simulink model "MBE_Simulation_04_Template_14_11_final"  (R2017b)
settings: Solver=FixedStepAuto  StartTime=0.0  StopTime=inf  FixedStep=0.05  RelTol=1e-3
libraries: simulink x67, canmsglib x4, instrumentlib x2, realtime_pacer_lib x1, hdlsllib x1
(part 3 of 4)

== system MBE_Simulation_04_Template_14_11_final/LeuchtenBlinkerBox/LB_Box_Simulation_Input/CanReceive_Cockpit_1 ==
  CanData_Cockpit_1_In : Inport
  Bus Selector : BusSelector  OutputSignals=CanData_Cockpit_1,CanTrigger_Cockpit_1
  Detect Change4 : simulink/Logic and Bit Operations/Detect Change  vinit=0  OutDataTypeStr=boolean
  Terminator6 : Terminator
  CanData_Cockpit_1_Out : Outport
  CanTrigger_Cockpit_1_Out : Outport  Port=2
  wires:
  Bus Selector/1 -> CanData_Cockpit_1_Out/1, Detect Change4/1  "<CanData_Cockpit_1>"
  Bus Selector/2 -> Terminator6/1  "<CanTrigger_Cockpit_1>"
  CanData_Cockpit_1_In/1 -> Bus Selector/1
  Detect Change4/1 -> CanTrigger_Cockpit_1_Out/1

== system MBE_Simulation_04_Template_14_11_final/LeuchtenBlinkerBox/LB_Box_Simulation_Input/CanReceive_Schloss_1 ==
  CanMsg_Schloss_1_In : Inport
  Bus Selector4 : BusSelector  OutputSignals=CanData_Schloss_1,CanTrigger_Schloss_1
  Detect Change4 : simulink/Logic and Bit Operations/Detect Change  vinit=0  OutDataTypeStr=boolean
  Terminator4 : Terminator
  CanData_Schloss_1_Out : Outport
  CanTrigger_Schloss_1_Out : Outport  Port=2
  wires:
  Bus Selector4/2 -> Terminator4/1  "<CanTrigger_Schloss_1>"
  CanMsg_Schloss_1_In/1 -> Bus Selector4/1
  Bus Selector4/1 -> Detect Change4/1, CanData_Schloss_1_Out/1  "<CanData_Schloss_1>"
  Detect Change4/1 -> CanTrigger_Schloss_1_Out/1

== system MBE_Simulation_04_Template_14_11_final/LeuchtenBlinkerBox/LB_Box_Simulation_Input/CanReceive_Sensor_1 ==
  CanMsg_Sensor_1_In : Inport
  Bus Selector2 : BusSelector  OutputSignals=CanData_Sensor_1,CanTrigger_Sensor_1
  CanData_Sensor_1_Out : Outport
  CanTrigger_Sensor_1_Out : Outport  Port=2
  wires:
  Bus Selector2/1 -> CanData_Sensor_1_Out/1  "<CanData_Sensor_1>"
  CanMsg_Sensor_1_In/1 -> Bus Selector2/1
  Bus Selector2/2 -> CanTrigger_Sensor_1_Out/1  "<CanTrigger_Sensor_1>"

== system MBE_Simulation_04_Template_14_11_final/LeuchtenBlinkerBox/LB_Box_Simulation_Input/GuiInput_LichtBox ==
  Bus Selector : BusSelector  OutputSignals=lightGenericButton
  GenericButton_Out : Outport
  wires:
  [lightInputBus] -> Bus Selector/1
  Bus Selector/1 -> GenericButton_Out/1  "<lightGenericButton>"

== system MBE_Simulation_04_Template_14_11_final/LeuchtenBlinkerBox/LB_Box_Simulation_Output/LeuchtenBlinkerLEDs ==
  FEL_LED : Inport  OutDataTypeStr=boolean
  ABL_LED : Inport  Port=2  OutDataTypeStr=boolean
  TFL_LED : Inport  Port=3  OutDataTypeStr=boolean
  BLL_LED : Inport  Port=4  OutDataTypeStr=boolean
  BLR_LED : Inport  Port=5  OutDataTypeStr=boolean
  BRL_LED : Inport  Port=6  OutDataTypeStr=boolean
  Terminator{,1..5} (6 alike) : Terminator
  wires:
  BLR_LED/1 -> Terminator1/1
  ABL_LED/1 -> Terminator3/1
  TFL_LED/1 -> Terminator2/1
  BLL_LED/1 -> Terminator/1
  FEL_LED/1 -> Terminator4/1
  BRL_LED/1 -> Terminator5/1

== system MBE_Simulation_04_Template_14_11_final/MLF-VirtualPlatform Setup/Subsystem/Triggered Subsystem ==
  outputAlarmSignals : Inport
  "outputLightSignals " : Inport  Port=2  OutDataTypeStr=boolean
  outputWindshieldSignals : Inport  Port=3  OutDataTypeStr=boolean
  Trigger : TriggerPort  TriggerType=falling  VariantControl=Variant
  Bus Selector : BusSelector  OutputSignals=lightUpperBeamHeadlight,lightReverselight,lightLowerBeamHeadlight,lightIndicatorRight,lightIndicatorLeft,lightGenericLightUp,lightGenericLightRight,lightGenericLightLeft,lightGenericLightDown,lightFoglightRight,lightFoglightLeft,lightDaylight,lightBrakelight,lightBacklight
  Bus Selector1 : BusSelector  OutputSignals=alarmLockLight,alarmGenericLightUp,alarmGenericLightRight,alarmGenericLightLeft,alarmGenericLightDown,alarmAlarmLight
  Bus Selector2 : BusSelector  OutputSignals=windshieldWiperD,windshieldWiperC,windshieldWiperB,windshieldWiperA,windshieldWasherPump,windshieldHeater,windshieldGenericLightUp,windshieldGenericLightRight,windshieldGenericLightLeft,windshieldGenericLightDown
  MATLAB Function : MATLAB Function  TreatAsAtomicUnit=on
  MATLAB Function1 : MATLAB Function  Commented=on  TreatAsAtomicUnit=on
  UDP Send : instrumentlib/UDP Send  Host=127.0.0.1  Port=50000  LocalPort=-1  EnableBlockingMode=off  ByteOrder=BigEndian
      settings: SourceProductName=Instrument Control Toolbox
  wires:
  "outputLightSignals "/1 -> Bus Selector/1
  outputAlarmSignals/1 -> Bus Selector1/1
  Bus Selector1/6 -> MATLAB Function/1(alarmAlarmLight)  "<alarmAlarmLight>"
  Bus Selector1/5 -> MATLAB Function/2(alarmGenericLightDown)  "<alarmGenericLightDown>"
  Bus Selector1/4 -> MATLAB Function/3(alarmGenericLightLeft)  "<alarmGenericLightLeft>"
  Bus Selector1/3 -> MATLAB Function/4(alarmGenericLightRight)  "<alarmGenericLightRight>"
  Bus Selector1/2 -> MATLAB Function/5(alarmGenericLightUp)  "<alarmGenericLightUp>"
  Bus Selector1/1 -> MATLAB Function/6(alarmLockLight)  "<alarmLockLight>"
  Bus Selector/14 -> MATLAB Function/7(lightBacklight)  "<lightBacklight>"
  Bus Selector/13 -> MATLAB Function/8(lightBrakelight)  "<lightBrakelight>"
  Bus Selector/12 -> MATLAB Function/9(lightDaylight)  "<lightDaylight>"
  Bus Selector/11 -> MATLAB Function/10(lightFoglightLeft)  "<lightFoglightLeft>"
  Bus Selector/9 -> MATLAB Function/12(lightGenericLightDown)  "<lightGenericLightDown>"
  Bus Selector/10 -> MATLAB Function/11(lightFoglightRight)  "<lightFoglightRight>"
  Bus Selector/8 -> MATLAB Function/13(lightGenericLightLeft)  "<lightGenericLightLeft>"
  Bus Selector/7 -> MATLAB Function/14(lightGenericLightRight)  "<lightGenericLightRight>"
  Bus Selector/6 -> MATLAB Function/15(lightGenericLightUp)  "<lightGenericLightUp>"
  Bus Selector/5 -> MATLAB Function/16(lightIndicatorLeft)  "<lightIndicatorLeft>"
  Bus Selector/4 -> MATLAB Function/17(lightIndicatorRight)  "<lightIndicatorRight>"
  Bus Selector/3 -> MATLAB Function/18(lightLowerBeamHeadlight)  "<lightLowerBeamHeadlight>"
  Bus Selector/2 -> MATLAB Function/19(lightReverselight)  "<lightReverselight>"
  Bus Selector/1 -> MATLAB Function/20(lightUpperBeamHeadlight)  "<lightUpperBeamHeadlight>"
  outputWindshieldSignals/1 -> Bus Selector2/1
  Bus Selector2/10 -> MATLAB Function/21(windshieldGenericLightDown)  "<windshieldGenericLightDown>"
  Bus Selector2/9 -> MATLAB Function/22(windshieldGenericLightLeft)  "<windshieldGenericLightLeft>"
  Bus Selector2/8 -> MATLAB Function/23(windshieldGenericLightRight)  "<windshieldGenericLightRight>"
  Bus Selector2/7 -> MATLAB Function/24(windshieldGenericLightUp)  "<windshieldGenericLightUp>"
  Bus Selector2/6 -> MATLAB Function/25(windshieldHeater)  "<windshieldHeater>"
  Bus Selector2/5 -> MATLAB Function/26(windshieldWasherPump)  "<windshieldWasherPump>"
  Bus Selector2/4 -> MATLAB Function/27(windshieldWiperA)  "<windshieldWiperA>"
  Bus Selector2/3 -> MATLAB Function/28(windshieldWiperB)  "<windshieldWiperB>"
  Bus Selector2/2 -> MATLAB Function/29(windshieldWiperC)  "<windshieldWiperC>"
  Bus Selector2/1 -> MATLAB Function/30(windshieldWiperD)  "<windshieldWiperD>"
  MATLAB Function/1(json_output) -> UDP Send/1

== system MBE_Simulation_04_Template_14_11_final/MLF-VirtualPlatform Setup/Subsystem2/Triggered Subsystem ==
  In1 : Inport
  Trigger : TriggerPort  VariantControl=Variant
  Bus Creator : BusCreator  Inputs=49
  MATLAB Function : MATLAB Function  TreatAsAtomicUnit=on
  outputAlarmSignals : Outport
  wires:
  In1/1 -> MATLAB Function/1(json_input)
  Bus Creator/1 -> outputAlarmSignals/1
  MATLAB Function/1(alarmAlarmButton) -> Bus Creator/1
  MATLAB Function/2(alarmAlarmLight) -> Bus Creator/2
  MATLAB Function/3(alarmGenericButton) -> Bus Creator/3
  MATLAB Function/4(alarmGenericLightDown) -> Bus Creator/4
  MATLAB Function/5(alarmGenericLightLeft) -> Bus Creator/5
  MATLAB Function/6(alarmGenericLightRight) -> Bus Creator/6
  MATLAB Function/7(alarmGenericLightUp) -> Bus Creator/7
  MATLAB Function/8(alarmLockButton) -> Bus Creator/8
  MATLAB Function/9(alarmLockLight) -> Bus Creator/9
  MATLAB Function/10(cockpitAlarmReset) -> Bus Creator/10
  MATLAB Function/11(cockpitBrake) -> Bus Creator/11
  MATLAB Function/13(cockpitIndicator) -> Bus Creator/13
  MATLAB Function/12(cockpitIgnition) -> Bus Creator/12
  MATLAB Function/14(cockpitLightSwitch) -> Bus Creator/14
  MATLAB Function/15(cockpitSteeringAngleDeg) -> Bus Creator/15
  MATLAB Function/16(cockpitTemperature) -> Bus Creator/16
  MATLAB Function/17(cockpitVelocity) -> Bus Creator/17
  MATLAB Function/18(cockpitWarnLight) -> Bus Creator/18
  MATLAB Function/19(cockpitWindshieldHeater) -> Bus Creator/19
  MATLAB Function/20(cockpitWindshieldWasherMode) -> Bus Creator/20
  MATLAB Function/21(cockpitWindshieldWasherPump) -> Bus Creator/21
  MATLAB Function/22(lightBacklight) -> Bus Creator/22
  MATLAB Function/23(lightBrakelight) -> Bus Creator/23
  MATLAB Function/24(lightDaylight) -> Bus Creator/24
  MATLAB Function/25(lightFoglightLeft) -> Bus Creator/25
  MATLAB Function/26(lightFoglightRight) -> Bus Creator/26
  MATLAB Function/27(lightGenericButton) -> Bus Creator/27
  MATLAB Function/29(lightGenericLightLeft) -> Bus Creator/29
  MATLAB Function/28(lightGenericLightDown) -> Bus Creator/28
  MATLAB Function/30(lightGenericLightRight) -> Bus Creator/30
  MATLAB Function/31(lightGenericLightUp) -> Bus Creator/31
  MATLAB Function/32(lightIndicatorLeft) -> Bus Creator/32
  MATLAB Function/33(lightIndicatorRight) -> Bus Creator/33
  MATLAB Function/34(lightLowerBeamHeadlight) -> Bus Creator/34
  MATLAB Function/35(lightReverselight) -> Bus Creator/35
  MATLAB Function/36(lightUpperBeamHeadlight) -> Bus Creator/36
  MATLAB Function/37(windshieldDistanceSensor) -> Bus Creator/37
  MATLAB Function/38(windshieldGenericButton) -> Bus Creator/38
  MATLAB Function/39(windshieldGenericLightDown) -> Bus Creator/39
  MATLAB Function/40(windshieldGenericLightLeft) -> Bus Creator/40
  MATLAB Function/41(windshieldGenericLightRight) -> Bus Creator/41
  MATLAB Function/42(windshieldGenericLightUp) -> Bus Creator/42
  MATLAB Function/43(windshieldHeater) -> Bus Creator/43
  MATLAB Function/44(windshieldLightSensor) -> Bus Creator/44
  MATLAB Function/45(windshieldWasherPump) -> Bus Creator/45
  MATLAB Function/46(windshieldWiperA) -> Bus Creator/46
  MATLAB Function/47(windshieldWiperB) -> Bus Creator/47
  MATLAB Function/48(windshieldWiperC) -> Bus Creator/48
  MATLAB Function/49(windshieldWiperD) -> Bus Creator/49

== system MBE_Simulation_04_Template_14_11_final/SchlossAlarmBox/SA_Box_Applikation/CanCoder_Alarm_1 ==
  AlarmZustand : Inport
  Bit Clear : simulink/Logic and Bit Operations/Bit Clear  iBit=0
      settings: SourceProductName=Simulink  SourceProductBaseCode=SL
  Bit Set : simulink/Logic and Bit Operations/Bit Set  iBit=0
      settings: SourceProductName=Simulink  SourceProductBaseCode=SL
  Data Type Conversion : DataTypeConversion  OutDataTypeStr=int16
  Detect Change : simulink/Logic and Bit Operations/Detect Change  vinit=0  OutDataTypeStr=boolean
  Scope : Scope
  Switch : Switch  Criteria=u2 ~= 0  Threshold=1
  CanData_Alarm_1 : Outport
  CanTrigger_Alarm_1 : Outport  Port=2
  wires:
  Data Type Conversion/1 -> Switch/2, Bit Clear/1, Bit Set/1
  Bit Set/1 -> Switch/1
  Bit Clear/1 -> Switch/3
  Switch/1 -> CanData_Alarm_1/1
  Detect Change/1 -> Scope/1, CanTrigger_Alarm_1/1
  AlarmZustand/1 -> Detect Change/1, Data Type Conversion/1

== system MBE_Simulation_04_Template_14_11_final/SchlossAlarmBox/SA_Box_Applikation/CanCoder_Schloss_1 ==
  SchliessZustand : Inport
  CAN Pack : canmsglib/CAN Pack  MsgList=(none)  MsgName=CAN Msg  MsgIDType=Standard (11-bit identifier)  MsgIdentifier=25  MsgLength=1  NSignals=0  StartBits=0  SignalSizes=0  ByteOrders=0  DataTypes=0  MultiplexTypes=0  MultiplexValues=0  Factors=0  Offsets=0  Minimums=0  Maximums=0  Remote=off  ApplyMinMax=off  BusOutput=off
      settings: SourceProductName=Simulink Real-Time  SourceProductBaseCode=XP  DataFormat=raw data
  CAN Pack1 : canmsglib/CAN Pack  MsgList=(none)  MsgName=CAN Msg  MsgIDType=Standard (11-bit identifier)  MsgIdentifier=25  MsgLength=8  NSignals=0  StartBits=0  SignalSizes=0  ByteOrders=0  DataTypes=0  MultiplexTypes=0  MultiplexValues=0  Factors=0  Offsets=0  Minimums=0  Maximums=0  Remote=off  ApplyMinMax=off  BusOutput=off
      settings: SourceProductName=Simulink Real-Time  SourceProductBaseCode=XP  DataFormat=raw data
  CAN Unpack : canmsglib/CAN Unpack  MsgList=(none)  MsgName=Data_Cockpit_1  MsgIDType=Standard (11-bit identifier)  MsgIdentifier=25  MsgLength=1  SignalInfo=SchlossZustand$0$1$1$2$1$0$1$0$-Inf$Inf$#  NSignals=1  IDPort=off  TimestampPort=off  ErrorPort=off  RemotePort=off  LengthPort=off  StatusPort=off  StartBits=str2num('[int32(0)]')  SignalSizes=str2num('[int32(1)]')  ByteOrders=str2num('[int32(1)]')  DataTypes=str2num('[int32(2)]')  MultiplexTypes=str2num('[int32(1)]')  MultiplexValues=str2num('[double(0)]')  Factors=str2num('[double(1)]')  Offsets=str2num('[double(0)]')  Minimums=str2num('[double(-Inf)]')  Maximums=str2num('[double(Inf)]')  ApplyMinMax=off
      settings: SourceProductName=Simulink Real-Time  SourceProductBaseCode=XP
  CAN Unpack1 : canmsglib/CAN Unpack  MsgList=(none)  MsgName=Data_Cockpit_1  MsgIDType=Standard (11-bit identifier)  MsgIdentifier=25  MsgLength=1  SignalInfo=SchlossTrigger$1$1$1$2$1$0$1$0$-Inf$Inf$#  NSignals=1  IDPort=off  TimestampPort=off  ErrorPort=off  RemotePort=off  LengthPort=off  StatusPort=off  StartBits=str2num('[int32(1)]')  SignalSizes=str2num('[int32(1)]')  ByteOrders=str2num('[int32(1)]')  DataTypes=str2num('[int32(2)]')  MultiplexTypes=str2num('[int32(1)]')  MultiplexValues=str2num('[double(0)]')  Factors=str2num('[double(1)]')  Offsets=str2num('[double(0)]')  Minimums=str2num('[double(-Inf)]')  Maximums=str2num('[double(Inf)]')  ApplyMinMax=off
      settings: SourceProductName=Simulink Real-Time  SourceProductBaseCode=XP
  Detect Change : simulink/Logic and Bit Operations/Detect Change  vinit=0  OutDataTypeStr=boolean
  CanData_Schloss_1 : Outport
  CanTrigger_Schloss_1 : Outport  Port=2
  wires:
  SchliessZustand/1 -> CAN Unpack/1, Detect Change/1
  Detect Change/1 -> CAN Unpack1/1
  CAN Unpack/1 -> CAN Pack/1
  CAN Unpack1/1 -> CAN Pack1/1
  CAN Pack/1 -> CanData_Schloss_1/1
  CAN Pack1/1 -> CanTrigger_Schloss_1/1

== system MBE_Simulation_04_Template_14_11_final/SchlossAlarmBox/SA_Box_Applikation/CanDecoder_Bremse_2 ==
  CanData_Bremse_2 : Inport
  Extract Bits : simulink/Logic and Bit Operations/Extract Bits  bitsToExtract=Range of bits  numBits=8  bitIdxRange=[0 7]  outScalingMode=Treat bit field as an integer
      settings: SourceProductName=Simulink
  Geschwindigkeit : Outport
  wires:
  CanData_Bremse_2/1 -> Extract Bits/1
  Extract Bits/1 -> Geschwindigkeit/1

== system MBE_Simulation_04_Template_14_11_final/SchlossAlarmBox/SA_Box_Applikation/CanDecoder_Cockpit_3 ==
  CanData_Cockpit_3 : Inport
  Compare To Zero : simulink/Logic and Bit Operations/Compare To Zero  relop=~=  OutDataTypeStr=boolean
  Extract Bits : simulink/Logic and Bit Operations/Extract Bits  bitsToExtract=Range of bits  numBits=8  bitIdxRange=[0 0]  outScalingMode=Treat bit field as an integer
      settings: SourceProductName=Simulink
  AlarmReset : Outport
  wires:
  CanData_Cockpit_3/1 -> Extract Bits/1
  Extract Bits/1 -> Compare To Zero/1
  Compare To Zero/1 -> AlarmReset/1

== system MBE_Simulation_04_Template_14_11_final/SchlossAlarmBox/SA_Box_Simulation_Input/CanBus_Input ==
  CanBus_SA_In : Inport
  Bus Selector2 : BusSelector  OutputSignals=CanBus_Cockpit.CanMsg_Cockpit_3,CanBus_Cockpit.CanMsg_Bremse_2
  CanMsg_Cockpit_3_Out : Outport
  CanMsg_Bremse_2_Out : Outport  Port=2
  wires:
  CanBus_SA_In/1 -> Bus Selector2/1
  Bus Selector2/1 -> CanMsg_Cockpit_3_Out/1  "<CanMsg_Cockpit_3>"
  Bus Selector2/2 -> CanMsg_Bremse_2_Out/1  "<CanMsg_Bremse_2>"

== system MBE_Simulation_04_Template_14_11_final/SchlossAlarmBox/SA_Box_Simulation_Input/CanReceive_Bremse_2 ==
  CanMsg_Bremse_2_In : Inport
  Bus Selector1 : BusSelector  OutputSignals=CanData_Bremse_2,CanTrigger_Bremse_2
  Detect Change4 : simulink/Logic and Bit Operations/Detect Change  vinit=0  OutDataTypeStr=boolean
  Terminator12 : Terminator
  CanData_Bremse_2_Out : Outport
  CanTrigger_Bremse_2_Out : Outport  Port=2
  wires:
  Bus Selector1/1 -> Detect Change4/1, CanData_Bremse_2_Out/1  "<CanData_Bremse_2>"
  Bus Selector1/2 -> Terminator12/1  "<CanTrigger_Bremse_2>"
  CanMsg_Bremse_2_In/1 -> Bus Selector1/1
  Detect Change4/1 -> CanTrigger_Bremse_2_Out/1

== system MBE_Simulation_04_Template_14_11_final/SchlossAlarmBox/SA_Box_Simulation_Input/CanReceive_Cockpit_3 ==
  CanMsg_Cockpit_3_In : Inport
  Bus Selector : BusSelector  OutputSignals=CanData_Cockpit_3,CanTrigger_Cockpit_3
  Detect Change4 : simulink/Logic and Bit Operations/Detect Change  vinit=0  OutDataTypeStr=boolean
  Terminator11 : Terminator
  CanData_Cockpit_3_Out : Outport
  CanTrigger_Cockpit_3_Out : Outport  Port=2
  wires:
  Bus Selector/1 -> Detect Change4/1, CanData_Cockpit_3_Out/1  "<CanData_Cockpit_3>"
  Bus Selector/2 -> Terminator11/1  "<CanTrigger_Cockpit_3>"
  CanMsg_Cockpit_3_In/1 -> Bus Selector/1
  Detect Change4/1 -> CanTrigger_Cockpit_3_Out/1

== system MBE_Simulation_04_Template_14_11_final/SchlossAlarmBox/SA_Box_Simulation_Input/PanelInput_SchlossAlarmBox ==
  AlarmButton : Constant  Value=0  OutDataTypeStr=uint8
  Bus Selector : BusSelector  OutputSignals=alarmGenericButton,alarmLockButton,alarmAlarmButton
  SchliessButton : Constant  Value=0  OutDataTypeStr=uint8
  Switch : Switch  Criteria=u2 > Threshold
  Switch1 : Switch  Criteria=u2 > Threshold
  GenericButton_Out : Outport
  SchliessButton_Out : Outport  Port=2
  AlarmButton_Out : Outport  Port=3
  wires:
  [alarmInputBus] -> Bus Selector/1
  Bus Selector/2 -> Switch/3  "<alarmLockButton>"
  Bus Selector/3 -> Switch1/3  "<alarmAlarmButton>"
  Bus Selector/1 -> GenericButton_Out/1  "<alarmGenericButton>"
  Switch/1 -> SchliessButton_Out/1
  Switch1/1 -> AlarmButton_Out/1
  [SwitchGUI] -> Switch1/2, Switch/2
  SchliessButton/1 -> Switch/1
  AlarmButton/1 -> Switch1/1

== system MBE_Simulation_04_Template_14_11_final/SchlossAlarmBox/SA_Box_Simulation_Output/CanBus_Output ==
  CanMsg_Alarm_1_In : Inport
  CanMsg_Schloss_1_In : Inport  Port=2
  Bus Creator1 : BusCreator  Inputs=2
  CanBus_SA_Out : Outport
  wires:
  CanMsg_Alarm_1_In/1 -> Bus Creator1/1
  CanMsg_Schloss_1_In/1 -> Bus Creator1/2
  Bus Creator1/1 -> CanBus_SA_Out/1  "CanBus_SA"

== system MBE_Simulation_04_Template_14_11_final/SchlossAlarmBox/SA_Box_Simulation_Output/CanTransmit_Alarm_1 ==
  CanData_Alarm_1_In : Inport
  CanTrigger_Alarm_1_In : Inport  Port=2
  Bus Creator : BusCreator  Inputs=2
  CanMsg_Alarm_1_Out : Outport
  wires:
  CanData_Alarm_1_In/1 -> Bus Creator/1
  CanTrigger_Alarm_1_In/1 -> Bus Creator/2
  Bus Creator/1 -> CanMsg_Alarm_1_Out/1  "CanMsg_Alarm_1"

== system MBE_Simulation_04_Template_14_11_final/SchlossAlarmBox/SA_Box_Simulation_Output/CanTransmit_Schloss_1 ==
  CanData_Schloss_1_In : Inport
  CanTrigger_Schloss_1_In : Inport  Port=2
  Bus Creator2 : BusCreator  Inputs=2
  CanMsg_Schloss_1_Out : Outport
  wires:
  CanTrigger_Schloss_1_In/1 -> Bus Creator2/2
  CanData_Schloss_1_In/1 -> Bus Creator2/1
  Bus Creator2/1 -> CanMsg_Schloss_1_Out/1  "CanMsg_Schloss_1"

== system MBE_Simulation_04_Template_14_11_final/SchlossAlarmBox/SA_Box_Simulation_Output/SchlossAlarmLEDs ==
  Schloss_LED : Inport
  Alarm_LED : Inport  Port=2
  Terminator : Terminator
  Terminator1 : Terminator
  wires:
  Schloss_LED/1 -> Terminator/1
  Alarm_LED/1 -> Terminator1/1

== system MBE_Simulation_04_Template_14_11_final/WischerSensorBox/WS_Box_Applikation/CanCoder_Sensor_1 ==
  Lichtsensor_In : Inport
  Distanzsensor_In : Inport  Port=2
  1-D Lookup Table : Lookup_n-D  NumberOfTableDimensions=1  BreakpointsForDimension1=[310,3800]  IndexSearchMethod=Linear search  Table=[500,0]  InternalRulePriority=Speed  RndMeth=Simplest  InputSameDT=on
  Bit Shift : hdlsllib/Logic and Bit Operations/Bit Shift  mode=Shift Left Logical  N=1
      settings: SourceProductName=Simulink
  Bitwise Operator : simulink/Logic and Bit Operations/Bitwise Operator  logicop=OR  UseBitMask=off  NumInputPorts=2  BitMask=bin2dec('11011001')  BitMaskRealWorld=Stored Integer
  Cast To Double : DataTypeConversion  OutDataTypeStr=double
  Data Type Conversion1 : DataTypeConversion  OutDataTypeStr=uint16
  Data Type Conversion2 : DataTypeConversion  OutDataTypeStr=uint16
  CanData_Sensor_1 : Outport
  wires:
  Distanzsensor_In/1 -> 1-D Lookup Table/1
  Lichtsensor_In/1 -> Data Type Conversion2/1
  1-D Lookup Table/1 -> Data Type Conversion1/1
  Data Type Conversion1/1 -> Bit Shift/1
  Bit Shift/1 -> Bitwise Operator/2
  Data Type Conversion2/1 -> Bitwise Operator/1
  Bitwise Operator/1 -> Cast To Double/1
  Cast To Double/1 -> CanData_Sensor_1/1

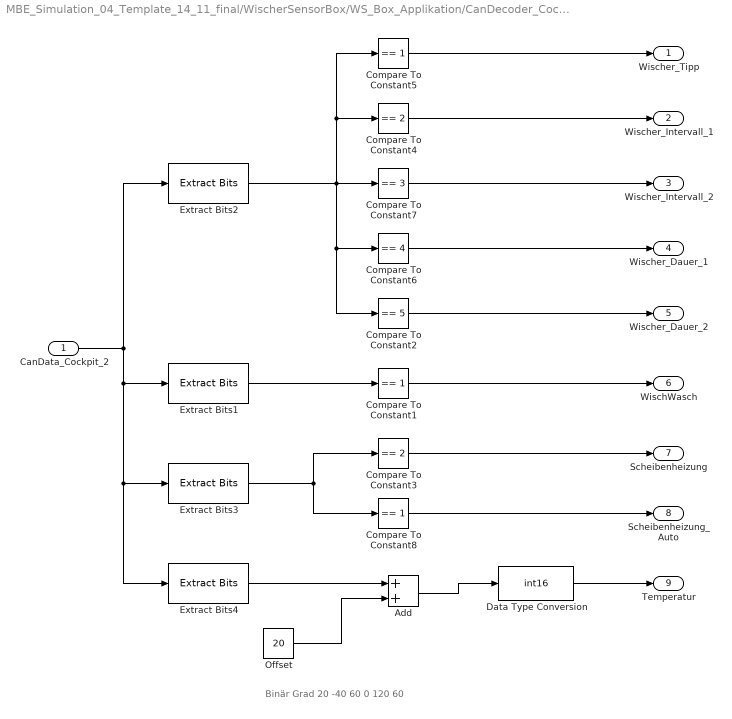
== system MBE_Simulation_04_Template_14_11_final/WischerSensorBox/WS_Box_Applikation/CanDecoder_Cockpit_2 ==
  note: Binär   Grad
      | 20		-40
      | 60		0
      | 120		60
  CanData_Cockpit_2 : Inport
  Add : Sum
  Compare To Constant1 : simulink/Logic and Bit Operations/Compare To Constant  relop===  const=1  OutDataTypeStr=boolean
  Compare To Constant2 : simulink/Logic and Bit Operations/Compare To Constant  relop===  const=5  OutDataTypeStr=boolean
  Compare To Constant3 : simulink/Logic and Bit Operations/Compare To Constant  relop===  const=2  OutDataTypeStr=boolean
  Compare To Constant4 : simulink/Logic and Bit Operations/Compare To Constant  relop===  const=2  OutDataTypeStr=boolean
  Compare To Constant5 : simulink/Logic and Bit Operations/Compare To Constant  relop===  const=1  OutDataTypeStr=boolean
  Compare To Constant6 : simulink/Logic and Bit Operations/Compare To Constant  relop===  const=4  OutDataTypeStr=boolean
  Compare To Constant7 : simulink/Logic and Bit Operations/Compare To Constant  relop===  const=3  OutDataTypeStr=boolean
  Compare To Constant8 : simulink/Logic and Bit Operations/Compare To Constant  relop===  const=1  OutDataTypeStr=boolean
  Data Type Conversion : DataTypeConversion  OutDataTypeStr=int16
  Extract Bits1 : simulink/Logic and Bit Operations/Extract Bits  bitsToExtract=Range of bits  numBits=8  bitIdxRange=[3 3]  outScalingMode=Treat bit field as an integer
      settings: SourceProductName=Simulink
  Extract Bits2 : simulink/Logic and Bit Operations/Extract Bits  bitsToExtract=Range of bits  numBits=8  bitIdxRange=[0 2]  outScalingMode=Treat bit field as an integer
      settings: SourceProductName=Simulink
  Extract Bits3 : simulink/Logic and Bit Operations/Extract Bits  bitsToExtract=Range of bits  numBits=8  bitIdxRange=[4 5]  outScalingMode=Treat bit field as an integer
      settings: SourceProductName=Simulink
  Extract Bits4 : simulink/Logic and Bit Operations/Extract Bits  bitsToExtract=Range of bits  numBits=8  bitIdxRange=[6 12]  outScalingMode=Treat bit field as an integer
      settings: SourceProductName=Simulink
  Offset : Constant  Value=20
  Wischer_Tipp : Outport
  Wischer_Intervall_1 : Outport  Port=2
  Wischer_Intervall_2 : Outport  Port=3
  Wischer_Dauer_1 : Outport  Port=4
  Wischer_Dauer_2 : Outport  Port=5
  WischWasch : Outport  Port=6
  Scheibenheizung : Outport  Port=7
  Scheibenheizung_Auto : Outport  Port=8
  Temperatur : Outport  Port=9
  wires:
  Extract Bits2/1 -> Compare To Constant5/1, Compare To Constant4/1, Compare To Constant2/1, Compare To Constant6/1, Compare To Constant7/1
  Compare To Constant5/1 -> Wischer_Tipp/1
  Compare To Constant4/1 -> Wischer_Intervall_1/1
  Compare To Constant7/1 -> Wischer_Intervall_2/1
  Compare To Constant6/1 -> Wischer_Dauer_1/1
  Compare To Constant2/1 -> Wischer_Dauer_2/1
  CanData_Cockpit_2/1 -> Extract Bits2/1, Extract Bits4/1, Extract Bits3/1, Extract Bits1/1
  Compare To Constant1/1 -> WischWasch/1
  Extract Bits1/1 -> Compare To Constant1/1
  Compare To Constant3/1 -> Scheibenheizung/1
  Compare To Constant8/1 -> Scheibenheizung_Auto/1
  Extract Bits3/1 -> Compare To Constant3/1, Compare To Constant8/1
  Data Type Conversion/1 -> Temperatur/1
  Add/1 -> Data Type Conversion/1
  Extract Bits4/1 -> Add/1
  Offset/1 -> Add/2

== system MBE_Simulation_04_Template_14_11_final/WischerSensorBox/WS_Box_Applikation/TriggerPuls ==
  Gain : Gain  Gain=2^0  OutDataTypeStr=uint8
  Pulse Generator : DiscretePulseGenerator  PulseType=Time based  Period=0.2  PulseWidth=50
  Scope : Scope
  TriggerPuls_200ms : Outport
  wires:
  Pulse Generator/1 -> Gain/1
  Gain/1 -> TriggerPuls_200ms/1, Scope/1

== system MBE_Simulation_04_Template_14_11_final/WischerSensorBox/WS_Box_Simulation_Input/CanBus_Input ==
  CanBus_WS_In : Inport
  Bus Selector1 : BusSelector  OutputSignals=CanBus_Cockpit.CanMsg_Cockpit_2,CanBus_SA.CanMsg_Schloss_1,CanBus_Cockpit.CanMsg_Bremse_2
  CanMsg_Cockpit_2_Out : Outport
  CanMsg_Schloss_1_Out : Outport  Port=2
  CanMsg_Bremse_2_Out : Outport  Port=3
  wires:
  Bus Selector1/1 -> CanMsg_Cockpit_2_Out/1  "<CanMsg_Cockpit_2>"
  CanBus_WS_In/1 -> Bus Selector1/1
  Bus Selector1/2 -> CanMsg_Schloss_1_Out/1  "<CanMsg_Schloss_1>"
  Bus Selector1/3 -> CanMsg_Bremse_2_Out/1  "<CanMsg_Bremse_2>"

== system MBE_Simulation_04_Template_14_11_final/WischerSensorBox/WS_Box_Simulation_Input/CanReceive_Bremse_2 ==
  CanMsg_Bremse_2_In : Inport
  Bus Selector1 : BusSelector  OutputSignals=CanData_Bremse_2,CanTrigger_Bremse_2
  Detect Change4 : simulink/Logic and Bit Operations/Detect Change  vinit=0  OutDataTypeStr=boolean
  Terminator12 : Terminator
  CanData_Bremse_2_Out : Outport
  CanTrigger_Bremse_2_Out : Outport  Port=2
  wires:
  Bus Selector1/1 -> Detect Change4/1, CanData_Bremse_2_Out/1  "<CanData_Bremse_2>"
  Bus Selector1/2 -> Terminator12/1  "<CanTrigger_Bremse_2>"
  CanMsg_Bremse_2_In/1 -> Bus Selector1/1
  Detect Change4/1 -> CanTrigger_Bremse_2_Out/1

== system MBE_Simulation_04_Template_14_11_final/WischerSensorBox/WS_Box_Simulation_Input/CanReceive_Cockpit_2 ==
  CanMsg_Cockpit_2_In : Inport
  Bus Selector : BusSelector  OutputSignals=CanData_Cockpit_2,CanTrigger_Cockpit_2
  Detect Change4 : simulink/Logic and Bit Operations/Detect Change  vinit=0  OutDataTypeStr=boolean
  Terminator11 : Terminator
  CanData_Cockpit_2_out : Outport
  CanTrigger_Cockpit_2_Out : Outport  Port=2
  wires:
  Bus Selector/2 -> Terminator11/1  "<CanTrigger_Cockpit_2>"
  CanMsg_Cockpit_2_In/1 -> Bus Selector/1
  Bus Selector/1 -> Detect Change4/1, CanData_Cockpit_2_out/1  "<CanData_Cockpit_2>"
  Detect Change4/1 -> CanTrigger_Cockpit_2_Out/1

== system MBE_Simulation_04_Template_14_11_final/WischerSensorBox/WS_Box_Simulation_Input/CanReceive_Schloss_1 ==
  CanMsg_Schloss_1_In : Inport
  Bus Selector4 : BusSelector  OutputSignals=CanData_Schloss_1,CanTrigger_Schloss_1
  Detect Change4 : simulink/Logic and Bit Operations/Detect Change  vinit=0  OutDataTypeStr=boolean
  Terminator4 : Terminator
  CanData_Schloss_1_Out : Outport
  CanTrigger_Schloss_1_Out : Outport  Port=2
  wires:
  Bus Selector4/2 -> Terminator4/1  "<CanTrigger_Schloss_1>"
  CanMsg_Schloss_1_In/1 -> Bus Selector4/1
  Bus Selector4/1 -> Detect Change4/1, CanData_Schloss_1_Out/1  "<CanData_Schloss_1>"
  Detect Change4/1 -> CanTrigger_Schloss_1_Out/1

== system MBE_Simulation_04_Template_14_11_final/WischerSensorBox/WS_Box_Simulation_Input/PanelInput_WischerSensorBox ==
  Bus Selector : BusSelector  OutputSignals=windshieldGenericButton,windshieldLightSensor,windshieldDistanceSensor
  DistanzSlider : Constant  Value=1779.8095238095  OutDataTypeStr=uint16
  LichtSwitch : Constant  Value=0  OutDataTypeStr=uint8
  Switch1 : Switch  Criteria=u2 > Threshold
  Switch13 : Switch  Criteria=u2 > Threshold
  GenericButton_Out : Outport
  LichtSwitch_Out : Outport  Port=2
  DistanzSlider_Out : Outport  Port=3
  wires:
  [windshieldInputBus] -> Bus Selector/1
  Bus Selector/1 -> GenericButton_Out/1  "<windshieldGenericButton>"
  Bus Selector/2 -> Switch13/3  "<windshieldLightSensor>"
  Bus Selector/3 -> Switch1/3  "<windshieldDistanceSensor>"
  Switch13/1 -> LichtSwitch_Out/1
  Switch1/1 -> DistanzSlider_Out/1
  [SwitchGUI] -> Switch1/2, Switch13/2
  LichtSwitch/1 -> Switch13/1
  DistanzSlider/1 -> Switch1/1

== system MBE_Simulation_04_Template_14_11_final/WischerSensorBox/WS_Box_Simulation_Output/CanBus_Output ==
  CanMsg_Sensor_1_In : Inport
  Bus Creator1 : BusCreator  Inputs=1
  CanBus_WS_Out : Outport
  wires:
  CanMsg_Sensor_1_In/1 -> Bus Creator1/1
  Bus Creator1/1 -> CanBus_WS_Out/1  "CanBus_WS"

== system MBE_Simulation_04_Template_14_11_final/WischerSensorBox/WS_Box_Simulation_Output/CanTransmit_Sensor_1 ==
  CanData_Sensor_1_In : Inport
  CanTrigger_Sensor_1_In : Inport  Port=2
  Bus Creator : BusCreator  Inputs=2
  OutCanMsg_Sensor_1_Out : Outport
  wires:
  CanData_Sensor_1_In/1 -> Bus Creator/1
  CanTrigger_Sensor_1_In/1 -> Bus Creator/2
  Bus Creator/1 -> OutCanMsg_Sensor_1_Out/1  "CanMsg_Sensor_1"

== system MBE_Simulation_04_Template_14_11_final/WischerSensorBox/WS_Box_Simulation_Output/Schrittmotor ==
  SM_A : Inport  OutDataTypeStr=boolean
  SM_B : Inport  Port=2  OutDataTypeStr=boolean
  SM_C : Inport  Port=3  OutDataTypeStr=boolean
  SM_D : Inport  Port=4  OutDataTypeStr=boolean
  Terminator{3..6} (4 alike) : Terminator
  wires:
  SM_C/1 -> Terminator5/1
  SM_D/1 -> Terminator6/1
  SM_A/1 -> Terminator3/1
  SM_B/1 -> Terminator4/1

== system MBE_Simulation_04_Template_14_11_final/WischerSensorBox/WS_Box_Simulation_Output/WischerSensorLEDs ==
  WW_LED : Inport  OutDataTypeStr=boolean
  SH_LED : Inport  Port=2  OutDataTypeStr=boolean
  Terminator3 : Terminator
  Terminator4 : Terminator
  wires:
  SH_LED/1 -> Terminator4/1
  WW_LED/1 -> Terminator3/1

== stateflow chart MBE_Simulation_04_Template_14_11_final/LeuchtenBlinkerBox/LB_Box_Applikation/Steuerung_Licht ==
  state State_Licht_ABL
    entry:
    FEL_LED=false;
    ABL_LED=true;
    TFL_LED=false;
    RL_LED = true
  state State_Licht_Auto
    state Dunkel
      entry: RL_LED = true
      state Gegenverkehr_nein
        entry:
        FEL_LED=true;
        ABL_LED=false;
        TFL_LED=false;
      state Gegenverkehr_Ja
        entry:
        FEL_LED=false;
        ABL_LED=true;
        TFL_LED=false;
      Gegenverkehr_nein -> Gegenverkehr_Ja : [Distanz < 250]
      Gegenverkehr_Ja -> Gegenverkehr_nein : [Distanz > 250]
      (default) -> Gegenverkehr_Ja
    state Hell
      entry:
      FEL_LED = false;
      ABL_LED = false;
      TFL_LED = true;
      RL_LED = false
    (default) -> Hell
    Hell -> Dunkel : [Helligkeit == 1]
    Dunkel -> Hell : [Helligkeit == 0]
  state State_OFF
    entry:
    FEL_LED=false;
    ABL_LED=false;
    TFL_LED=false;
  state State_Licht_FEL
    entry:
    FEL_LED=true;
    ABL_LED=false;
    TFL_LED=false;
    RL_LED = true
  state State_Licht_TFL
    entry:
    FEL_LED=false;
    ABL_LED=false;
    TFL_LED=true;
    RL_LED = false
  State_Licht_ABL -> State_OFF : [Licht_ABL == 0]
  State_OFF -> State_Licht_ABL [order 1] : [Licht_ABL == 1]
  (default) -> State_OFF
  State_OFF -> State_Licht_FEL [order 2] : [Licht_FEL == 1]
  State_Licht_Auto -> State_OFF : [Licht_Auto == 0]
  State_OFF -> State_Licht_Auto [order 4] : [Licht_Auto==1]
  State_Licht_FEL -> State_OFF : [Licht_FEL==0]
  State_OFF -> State_Licht_TFL [order 3] : [Licht_TFL==1]
  State_Licht_TFL -> State_OFF : [Licht_TFL== 0]
  data: FEL_LED output boolean; Helligkeit input boolean; Distanz input uint16; ABL_LED output boolean; TFL_LED output boolean; Licht_Auto input boolean; Licht_TFL input boolean; Licht_ABL input boolean; Licht_FEL input boolean; RL_LED output boolean

== stateflow chart MBE_Simulation_04_Template_14_11_final/SchlossAlarmBox/SA_Box_Applikation/Chart ==
  state State_Geschlossen
    en, du: SchliessZustand = true
    state State_AA_OFF
    state State_AA_ON
      state State_TRIGGER_ON
        en, du: AlarmZustand = true
        AlarmLED = true
      state State_TRIGGER_OFF
        state State_AlarmLED_OFF
          en, du: AlarmLED = false
        state State_AlarmLED_ON
          en, du: AlarmLED = true
        State_AlarmLED_OFF -> State_AlarmLED_ON : [after(0.5, sec)]
        (default) -> State_AlarmLED_ON
        State_AlarmLED_ON -> State_AlarmLED_OFF : [AlarmZustand == false && after(0.5, sec)]
      State_TRIGGER_OFF -> State_TRIGGER_ON : [AlarmButton == true]
      (default) -> State_TRIGGER_OFF
    (default) -> State_AA_OFF
    State_AA_OFF -> State_AA_ON : [Geschwindigkeit == 0]
    State_AA_ON -> State_AA_OFF : [Geschwindigkeit > 0]
  state State_Offen
    en, du: SchliessZustand = false
    state State_AlarmReset_Gedrueckt
      en, du: AlarmZustand = false
      AlarmLED = false
    state State_AlarmReset_NichtGedrueckt
    State_AlarmReset_NichtGedrueckt -> State_AlarmReset_Gedrueckt : [AlarmReset == true]
    (default) -> State_AlarmReset_NichtGedrueckt
  (default) -> State_Offen : {AlarmZustand = false}
  State_Offen -> State_Geschlossen : [SchliessButton == true && after(0.5,sec)]
  State_Geschlossen -> State_Offen [order 2] : [SchliessButton == true && after(0.5,sec)]
  State_Geschlossen -> State_Offen [order 1] : [SchliessButton == true && AlarmZustand == false && after(0.5,sec)]{AlarmLED = false}
  data: SchliessButton input; AlarmButton input; SchliessZustand output boolean; AlarmZustand output boolean; AlarmReset input; Geschwindigkeit input; AlarmLED output boolean; AlarmResetTriggered input boolean
  events: AlarmResetUpdated local FUNCTION_CALL_EVENT

== stateflow chart MBE_Simulation_04_Template_14_11_final/LeuchtenBlinkerBox/LB_Box_Applikation/Steuerung_Blinker ==
  state State_Blinker_Bedienung
    state State_OFF
      en, du:
      Blinker_Aktiv = false
    state State_Blinken_Rechts
      en, du:
      Rechte_Seite_an = true
      Linke_Seite_an = false
      Blink_Frequenz =0.5
      Blinker_Aktiv = true
    state State_Blinken_Links
      en, du:
      Rechte_Seite_an = false
      Linke_Seite_an = true
      Blink_Frequenz =0.5
      Blinker_Aktiv = true
    state State_Warnblinken
      en, du:
      Rechte_Seite_an = true
      Linke_Seite_an = true
      Blink_Frequenz =0.5
      Blinker_Aktiv = true
    state State_Alarmblinken
      en, du:
      Rechte_Seite_an = true
      Linke_Seite_an = true
      Blink_Frequenz =0.25
      Blinker_Aktiv = true
    state State_Komfort_Links
      en, du:
      Rechte_Seite_an = false
      Linke_Seite_an = true
      Blink_Frequenz =0.5
      Blinker_Aktiv = true
      blink_count = 2
      flag = true
    state State_Komfort_Rechts
      en, du:
      Rechte_Seite_an = true
      Linke_Seite_an = false
      Blink_Frequenz =0.5
      Blinker_Aktiv = true
      blink_count = 2
      flag = false
    state State_Blinker_Oeffnen_Schliessen
      en, du: Rechte_Seite_an = true
      Linke_Seite_an = true
      Blink_Frequenz =0.5
      if SchliessZustand == true
      blink_count = 1
      end
      Blinker_Aktiv = true
    (junction 202) -> State_OFF [order 8]
    (junction 202) -> State_Blinken_Rechts [order 3] : [Blinker_R]
    (junction 202) -> State_Blinken_Links [order 4] : [Blinker_L]
    (default) -> (junction 202)
    State_Blinker_Bedienung -> (junction 202) [order 1]
    (junction 202) -> State_Warnblinken [order 1] : [Warnblinker]
    (junction 202) -> State_Alarmblinken [order 2] : [AlarmZustand]
    (junction 202) -> State_Komfort_Links [order 5] : [Blinker_Tip_L]
    (junction 202) -> State_Komfort_Rechts [order 6] : [Blinker_Tip_R]
    (junction 202) -> State_Blinker_Oeffnen_Schliessen [order 7] : [SchliessZustandTriggered]
  state State_Blinker_ON
    en, du:
    BLL_LED=Linke_Seite_an
    BLR_LED=Rechte_Seite_an
  state State_Blinker_OFF
    en, du:
    BLL_LED=false
    BLR_LED=false
    if flag == true
    BlinkerLinks = true
    end
    if flag == false
    BlinkerRechts = true
    end
  (default) -> State_Blinker_Bedienung : {Blinker_Aktiv =false, BlinkerLinks = false, BlinkerRechts = false, flag = false, blink_count = 0}
  State_Blinker_ON -> State_Blinker_Bedienung [order 1] : [(Warnblinker || Blinker_L || Blinker_R) && blink_count > 0]{blink_count = 0, BlinkerLinks = false, BlinkerRechts = false}
  State_Blinker_OFF -> State_Blinker_ON [order 2] : [blink_count > 0 && after(Blink_Frequenz, sec)]{blink_count = blink_count - 1}
  State_Blinker_Bedienung -> State_Blinker_ON [order 1] : [Blinker_Aktiv == true]
  State_Blinker_ON -> State_Blinker_OFF [order 2] : [ after(Blink_Frequenz,sec)]
  State_Blinker_OFF -> State_Blinker_Bedienung [order 3] : [after(Blink_Frequenz, sec)]{BlinkerLinks = false, BlinkerRechts = false}
  State_Blinker_OFF -> State_Blinker_Bedienung [order 1] : [(Warnblinker || Blinker_L || Blinker_R || (BlinkerLinks == true && Blinker_Tip_R) || (BlinkerRechts == true && Blinker_Tip_L) )  && blink_count > 0]{blink_count = 0, BlinkerLinks = false, BlinkerRechts = false}
  data: BLL_LED output boolean; BLR_LED output boolean; Blinker_Tip_R input; Blinker_R input; Blinker_Tip_L input; Blinker_L input; Warnblinker input boolean; SchliessZustand input boolean; AlarmZustand input boolean; Count local; OpeningCount local; ClosingCount local; Opening local; Closing local; blink_left local boolean; blink_right local boolean; blink_count local uint32; blink_delay local double; SchliessZustandTriggered input; AlarmZustandTriggered input; Blink_Frequenz local double; Blinker_Aktiv local boolean; Rechte_Seite_an local boolean; Linke_Seite_an local boolean; Blinker_Stopp local; BlinkCounter local; BlinkerLinks local boolean; BlinkerRechts local boolean; flag local boolean
  events: SchliessZustandUpdated local FUNCTION_CALL_EVENT; AlarmZustandUpdated local FUNCTION_CALL_EVENT

== matlab function MBE_Simulation_04_Template_14_11_final/MLF-VirtualPlatform Setup/Subsystem/Triggered Subsystem/MATLAB Function ==
  data: alarmAlarmLight input; alarmGenericLightDown input; alarmGenericLightLeft input; alarmGenericLightRight input; alarmGenericLightUp input; alarmLockLight input; lightBacklight input; lightBrakelight input; lightDaylight input; json_output output size=4096; lightFoglightLeft input; lightFoglightRight input; lightGenericLightDown input; lightGenericLightLeft input; lightGenericLightRight input; lightGenericLightUp input; lightIndicatorLeft input; lightIndicatorRight input; lightLowerBeamHeadlight input; lightReverselight input; lightUpperBeamHeadlight input; windshieldGenericLightDown input; windshieldGenericLightLeft input; windshieldGenericLightRight input; windshieldGenericLightUp input; windshieldHeater input; windshieldWasherPump input; windshieldWiperA input; windshieldWiperB input; windshieldWiperC input; windshieldWiperD input
function json_output = fcn( ...
    alarmAlarmLight, ...
    alarmGenericLightDown, ...
    alarmGenericLightLeft, ...
    alarmGenericLightRight, ...
    alarmGenericLightUp, ...
    alarmLockLight, ...
    lightBacklight, ...
    lightBrakelight, ...
    lightDaylight, ...
    lightFoglightLeft, ...
    lightFoglightRight, ...
    lightGenericLightDown, ...
    lightGenericLightLeft, ...
    lightGenericLightRight, ...
    lightGenericLightUp, ...
    lightIndicatorLeft, ...
    lightIndicatorRight, ...
    lightLowerBeamHeadlight, ...
    lightReverselight, ...
    lightUpperBeamHeadlight, ...
    windshieldGenericLightDown, ...
    windshieldGenericLightLeft, ...
    windshieldGenericLightRight, ...
    windshieldGenericLightUp, ...
    windshieldHeater, ...
    windshieldWasherPump, ...
    windshieldWiperA, ...
    windshieldWiperB, ...
    windshieldWiperC, ...
    windshieldWiperD)

coder.extrinsic('jsonencode');

% Allocate output array size an initialize with zeroes
json_output = zeros(4096,1,'uint8');


% Prepare the data
json_struct = struct(...
    'alarmAlarmLight', alarmAlarmLight, ...
    'alarmGenericLightDown', alarmGenericLightDown, ...
    'alarmGenericLightLeft', alarmGenericLightLeft, ...
    'alarmGenericLightRight', alarmGenericLightRight, ...
    'alarmGenericLightUp', alarmGenericLightUp, ...
    'alarmLockLight', alarmLockLight, ...
    'lightBacklight',lightBacklight, ...
    'lightBrakelight',lightBrakelight, ...
    'lightDaylight',lightDaylight, ...
    'lightFoglightLeft', lightFoglightLeft, ...
    'lightFoglightRight', lightFoglightRight, ...
    'lightGenericLightDown', lightGenericLightDown, ...
    'lightGenericLightLeft', lightGenericLightLeft, ...
    'lightGenericLightRight', lightGenericLightRight, ...
    'lightGenericLightUp', lightGenericLightUp, ...
    'lightIndicatorLeft', lightIndicatorLeft, ...
    'lightIndicatorRight', lightIndicatorRight, ...
    'lightLowerBeamHeadlight', lightLowerBeamHeadlight, ...
    'lightReverselight', lightReverselight, ...
    'lightUpperBeamHeadlight', lightUpperBeamHeadlight, ...
    'windshieldGenericLightDown', windshieldGenericLightDown, ...
    'windshieldGenericLightLeft', windshieldGenericLightLeft, ...
    'windshieldGenericLightRight', windshieldGenericLightRight, ...
    'windshieldGenericLightUp', windshieldGenericLightUp, ...
    'windshieldHeater', windshieldHeater, ...
    'windshieldWasherPump', windshieldWasherPump, ...
    'windshieldWiperA', windshieldWiperA, ...
    'windshieldWiperB', windshieldWiperB, ...
    'windshieldWiperC', windshieldWiperC, ...
    'windshieldWiperD', windshieldWiperD ...
);

% Create json string from data
json_string = jsonencode(json_struct);

% Get length of final json string
len = uint16(0);
len = uint16(length(json_string));

% Copy json string char by char to output string
for i = 1:len
    json_output(i) = uint8(json_string(i));
end

json_output(len+1) = uint8(10);
